simulink model "Demo_veDYNA_cs"  (Simulink 7.6)
settings: Solver=ode1  SolverMode=SingleTasking  StartTime=0  StopTime=15  FixedStep=1/500  RelTol=1e-3
PreLoadFcn:
  | PreScanveDYNAPreLoadFcn(bdroot);
  | check_NUTS_defined;
  | 
  | assignin('base',['model_closed_' bdroot],false);
PostLoadFcn:
  | PreScanveDYNAPostLoadFcn(bdroot);
  | 
InitFcn:
  | vdy_SetExternalInputSource('ManLongCtrl',1,'Brake','other');
  | vdy_SetExternalInputSource('ManLongCtrl',1,'EngineTorque','other');
  | vdy_SetExternalInputSource('ManLatCtrl',1,'Steering','other');
  | 
  | PreScanveDYNAInitFcn(bdroot);
  | PreScanExperimentInitFcn(bdroot)
StopFcn:
  | PreScanExperimentStopFcn(bdroot)
undefined symbols (not defined in the file): at_period, CPT, DiscIntNeverNeededParam, vm_at_pulsewidth, vm_driver_dflt_gain, x_ini_VRML, y_ini_VRML, z_ini_VRML
libraries: dyna_cpt_lib x93, PreScanSimulinkLibrary x10, PreScanUsefulBlocks x4, simulink x4, anilib x3, dyna_lib x3, simulink_extras x2, dyna_manctrl_lib x2, dyna_road_lib x2, dyna_io_lib x1, dyna_demo_lib x1, dyna_usr_maneuver_states_lib x1
(part 5 of 8)

== system Demo_veDYNA_cs/Mazda_RX8_1/Simple ACC/Engine Torque Control/Demux Vehicle Info/gear_ratio ==
  RStatF : Inport
  GearRatioF : Inport  Port=2
  RStatR : Inport  Port=3
  GearRatioR : Inport  Port=4
  Product1 : Product  Inputs=/*  SaturateOnIntegerOverflow=on  InputSameDT=on  OutDataTypeStr=Inherit: Same as first input
  Product2 : Product  Inputs=/*  SaturateOnIntegerOverflow=on  InputSameDT=on  OutDataTypeStr=Inherit: Same as first input
  Sum : Sum  Inputs=|++  SaturateOnIntegerOverflow=on  InputSameDT=on  OutDataTypeStr=Inherit: Same as first input
  GearRatio : Outport
  wires:
  Sum/1 -> GearRatio/1
  Product2/1 -> Sum/1
  Product1/1 -> Sum/2
  RStatF/1 -> Product2/1
  GearRatioF/1 -> Product2/2
  RStatR/1 -> Product1/1
  GearRatioR/1 -> Product1/2

== system Demo_veDYNA_cs/Mazda_RX8_1/Simple ACC/Engine Torque Control/Demux Vehicle Info/mmot diff ==
  vIst : Inport
  gear_ratio : Inport  Port=2
  Theta : Inport  Port=3
  Theta Mot : Inport  Port=4
  vSoll : Inport  Port=5
  Product : Product  Inputs=3  SaturateOnIntegerOverflow=on  InputSameDT=on  OutDataTypeStr=Inherit: Same as first input
  Sum : Sum  Inputs=|++  SaturateOnIntegerOverflow=on  InputSameDT=on  OutDataTypeStr=Inherit: Same as first input
  Sum1 : Sum  Inputs=+-  SaturateOnIntegerOverflow=on  InputSameDT=on  OutDataTypeStr=Inherit: Same as first input
  Out1 : Outport
  wires:
  Product/1 -> Out1/1
  Sum1/1 -> Product/1
  Sum/1 -> Product/3
  gear_ratio/1 -> Product/2
  vSoll/1 -> Sum1/1
  vIst/1 -> Sum1/2
  Theta/1 -> Sum/1
  Theta Mot/1 -> Sum/2

== system Demo_veDYNA_cs/Mazda_RX8_1/Simple ACC/Engine Torque Control/Demux Vehicle Info/theta_red ==
  gear ratio : Inport
  VehMass : Inport  Port=2
  Constant : Constant
  Math Function : Math  Operator=square  SaturateOnIntegerOverflow=on
  Product1 : Product  Inputs=/*  SaturateOnIntegerOverflow=on  InputSameDT=on  OutDataTypeStr=Inherit: Same as first input
  Sum : Sum  Inputs=++|  SaturateOnIntegerOverflow=on  InputSameDT=on  OutDataTypeStr=Inherit: Same as first input
  Theta : Outport
  wires:
  Constant/1 -> Sum/1
  Sum/1 -> Product1/1
  Math Function/1 -> Sum/2
  gear ratio/1 -> Math Function/1
  Product1/1 -> Theta/1
  VehMass/1 -> Product1/2

== system Demo_veDYNA_cs/Nissan_Cabstar_1/Trajectories/Traj2State1/Traj2State2/MuxState ==
  x [m] : Inport
  y [m] : Inport  Port=2
  z [m] : Inport  Port=3
  dx [m/s] : Inport  Port=4
  dy [m/s] : Inport  Port=5
  dz [m/s] : Inport  Port=6
  R [rad] : Inport  Port=7
  P [rad] : Inport  Port=8
  Y [rad] : Inport  Port=9
  Mux : Mux  Inputs=9
  state : Outport
  wires:
  z [m]/1 -> Mux/3
  y [m]/1 -> Mux/2
  x [m]/1 -> Mux/1
  Y [rad]/1 -> Mux/9
  P [rad]/1 -> Mux/8
  R [rad]/1 -> Mux/7
  dz [m/s]/1 -> Mux/6
  dy [m/s]/1 -> Mux/5
  dx [m/s]/1 -> Mux/4
  Mux/1 -> state/1

== system Demo_veDYNA_cs/Nissan_Cabstar_1/Trajectories/Traj2State1/Traj2State2/Traj2MuxState_Ext ==
  Traj : Inport
  Terminator{1..9} (9 alike) : Terminator
  demux : Subsystem
  x [m] : Outport
  y [m] : Outport  Port=2
  z [m] : Outport  Port=3
  dx [m/s] : Outport  Port=4
  dy [m/s] : Outport  Port=5
  dz [m/s] : Outport  Port=6
  R [rad] : Outport  Port=7
  P [rad] : Outport  Port=8
  Y [rad] : Outport  Port=9
  wires:
  demux/9(Y) -> Y [rad]/1
  demux/7(R) -> R [rad]/1
  demux/5(vely) -> dy [m/s]/1
  demux/4(velx) -> dx [m/s]/1
  demux/10(velR) -> Terminator4/1
  demux/11(velP) -> Terminator5/1
  demux/12(velY) -> Terminator1/1
  demux/13(accx) -> Terminator8/1
  demux/14(accy) -> Terminator9/1
  demux/15(accz) -> Terminator7/1
  demux/18(accY) -> Terminator2/1
  demux/16(accR) -> Terminator3/1
  demux/17(accP) -> Terminator6/1
  demux/3(z) -> z [m]/1
  Traj/1 -> demux/1(traj)
  demux/6(velz) -> dz [m/s]/1
  demux/1(x) -> x [m]/1
  demux/2(y) -> y [m]/1
  demux/8(P) -> P [rad]/1

== system Demo_veDYNA_cs/Vedyna_Vehicle/CPT_MDL/MDL_PAR/BrkHyd/System Instance 1 ==
  pbrmaster [N/m**2] : Subsystem
      mask Display: disp('Master brake cylinder pressure [N/m**2]')

== system Demo_veDYNA_cs/Vedyna_Vehicle/CPT_MDL/MDL_PAR/ClutchCtrl/System Instance 1 ==
  Clutch [%] : Subsystem
      mask Display: disp('Clutch ratio [%]')

== system Demo_veDYNA_cs/Vedyna_Vehicle/CPT_MDL/MDL_PAR/Contact/System Instance 1 ==
  RoadZ [m] : Subsystem
      mask Display: disp('Local road excitation [m]')

== system Demo_veDYNA_cs/Vedyna_Vehicle/CPT_MDL/MDL_PAR/Contact/System Instance 2 ==
  RoadZ [m] : Subsystem
      mask Display: disp('Local road excitation [m]')

== system Demo_veDYNA_cs/Vedyna_Vehicle/CPT_MDL/MDL_PAR/Contact/System Instance 3 ==
  RoadZ [m] : Subsystem
      mask Display: disp('Local road excitation [m]')

== system Demo_veDYNA_cs/Vedyna_Vehicle/CPT_MDL/MDL_PAR/Contact/System Instance 4 ==
  RoadZ [m] : Subsystem
      mask Display: disp('Local road excitation [m]')

== system Demo_veDYNA_cs/Vedyna_Vehicle/CPT_MDL/MDL_PAR/Contact/System Instance 5 ==
  RoadZ [m] : Subsystem
      mask Display: disp('Local road excitation [m]')

== system Demo_veDYNA_cs/Vedyna_Vehicle/CPT_MDL/MDL_PAR/Contact/System Instance 6 ==
  RoadZ [m] : Subsystem
      mask Display: disp('Local road excitation [m]')

== system Demo_veDYNA_cs/Vedyna_Vehicle/CPT_MDL/MDL_PAR/Contact/System Instance 7 ==
  RoadZ [m] : Subsystem
      mask Display: disp('Local road excitation [m]')

== system Demo_veDYNA_cs/Vedyna_Vehicle/CPT_MDL/MDL_PAR/Contact/System Instance 8 ==
  RoadZ [m] : Subsystem
      mask Display: disp('Local road excitation [m]')

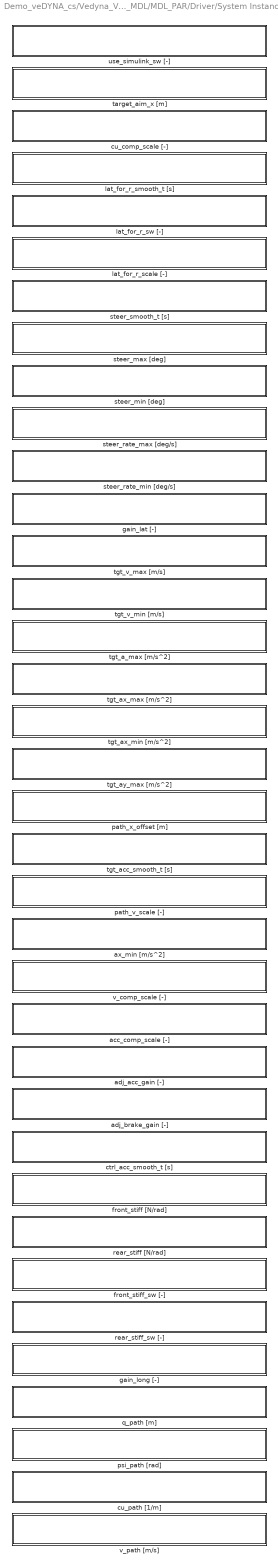
== system Demo_veDYNA_cs/Vedyna_Vehicle/CPT_MDL/MDL_PAR/Driver/System Instance 1 ==
  acc_comp_scale [-] : Subsystem
      mask Display: disp('v (acc_comp_scale) [-]')
  adj_acc_gain [-] : Subsystem
      mask Display: disp('v (adj_acc_gain) [-]')
  adj_brake_gain [-] : Subsystem
      mask Display: disp('v (adj_brake_gain) [-]')
  ax_min [m/s^2] : Subsystem
      mask Display: disp('v (ax_min) [m/s^2]')
  ctrl_acc_smooth_t [s] : Subsystem
      mask Display: disp('v (ctrl_acc_smooth_t) [s]')
  cu_comp_scale [-] : Subsystem
      mask Display: disp('v (cu_comp_scale) [-]')
  cu_path [1/m] : Subsystem
      mask Display: disp('path curvature [1/m]')
  front_stiff [N/rad] : Subsystem
      mask Display: disp('v (front_stiff) [N/rad]')
  front_stiff_sw [-] : Subsystem
      mask Display: disp('v (front_stiff_sw) [-]')
  gain_lat [-] : Subsystem
      mask Display: disp('v (gain_lat) [-]')
  gain_long [-] : Subsystem
      mask Display: disp('v (gain_long) [-]')
  lat_for_r_scale [-] : Subsystem
      mask Display: disp('v (lat_for_r_scale) [-]')
  lat_for_r_smooth_t [s] : Subsystem
      mask Display: disp('v (lat_for_r_smooth_t) [s]')
  lat_for_r_sw [-] : Subsystem
      mask Display: disp('v (lat_for_r_sw) [-]')
  path_v_scale [-] : Subsystem
      mask Display: disp('v (path_v_scale) [-]')
  path_x_offset [m] : Subsystem
      mask Display: disp('v (path_x_offset) [m]')
  psi_path [rad] : Subsystem
      mask Display: disp('path angle offset (relative to road''s center line) [rad]')
  q_path [m] : Subsystem
      mask Display: disp('lateral offset [m]')
  rear_stiff [N/rad] : Subsystem
      mask Display: disp('v (rear_stiff) [N/rad]')
  rear_stiff_sw [-] : Subsystem
      mask Display: disp('v (rear_stiff_sw) [-]')
  steer_max [deg] : Subsystem
      mask Display: disp('v (steer_max) [deg]')
  steer_min [deg] : Subsystem
      mask Display: disp('v (steer_min) [deg]')
  steer_rate_max [deg/s] : Subsystem
      mask Display: disp('v (steer_rate_max) [deg/s]')
  steer_rate_min [deg/s] : Subsystem
      mask Display: disp('v (steer_rate_min) [deg/s]')
  steer_smooth_t [s] : Subsystem
      mask Display: disp('v (steer_smooth_t) [s]')
  target_aim_x [m] : Subsystem
      mask Display: disp('v (target_aim_x) [m]')
  tgt_a_max [m/s^2] : Subsystem
      mask Display: disp('v (tgt_a_max) [m/s^2]')
  tgt_acc_smooth_t [s] : Subsystem
      mask Display: disp('v (tgt_acc_smooth_t) [s]')
  tgt_ax_max [m/s^2] : Subsystem
      mask Display: disp('v (tgt_ax_max) [m/s^2]')
  tgt_ax_min [m/s^2] : Subsystem
      mask Display: disp('v (tgt_ax_min) [m/s^2]')
  tgt_ay_max [m/s^2] : Subsystem
      mask Display: disp('v (tgt_ay_max) [m/s^2]')
  tgt_v_max [m/s] : Subsystem
      mask Display: disp('v (tgt_v_max) [m/s]')
  tgt_v_min [m/s] : Subsystem
      mask Display: disp('v (tgt_v_min) [m/s]')
  use_simulink_sw [-] : Subsystem
      mask Display: disp('v (use_simulink_sw) [-]')
  v_comp_scale [-] : Subsystem
      mask Display: disp('v (v_comp_scale) [-]')
  v_path [m/s] : Subsystem
      mask Display: disp('desired velocity [m/s]')

== system Demo_veDYNA_cs/Vedyna_Vehicle/CPT_MDL/MDL_PAR/Engine/System Instance 1 ==
  ASR_Flag [-] : Subsystem
      mask Display: disp('ASR Flag [-]')
  ASR_Torque [Nm] : Subsystem
      mask Display: disp('ASR Torque [Nm]')
  MSR_Flag [-] : Subsystem
      mask Display: disp('MSR Flag [-]')
  MSR_Torque [Nm] : Subsystem
      mask Display: disp('MSR Torque [Nm]')

== system Demo_veDYNA_cs/Vedyna_Vehicle/CPT_MDL/MDL_PAR/GearCtrl/System Instance 1 ==
  Gear [-] : Subsystem
      mask Display: disp('Gear position [-]')
  UpShiftRequest [-1,1] : Subsystem
      mask Display: disp('Up shift request [-1,1]')

== system Demo_veDYNA_cs/Vedyna_Vehicle/CPT_MDL/MDL_PAR/ManLatCtrl/System Instance 1 ==
  Curvature [1/m] : Subsystem
      mask Display: disp('Curvature [1/m]')
  Steering [deg] : Subsystem
      mask Display: disp('Steering wheel angle [deg]')

== system Demo_veDYNA_cs/Vedyna_Vehicle/CPT_MDL/MDL_PAR/ManLongCtrl/System Instance 1 ==
  AccelerationY [m/s**2] : Subsystem
      mask Display: disp('Lateral acceleration [m/s**2]')
  Brake [%] : Subsystem
      mask Display: disp('Brake position [%]')
  EngineTorque [Nm] : Subsystem
      mask Display: disp('Engine torque [Nm]')
  Speed [km/h] : Subsystem
      mask Display: disp('Speed [km/h]')
  Throttle [%] : Subsystem
      mask Display: disp('Throttle position [%]')

== system Demo_veDYNA_cs/Vedyna_Vehicle/CPT_MDL/MDL_PAR/Tmeasy/System Instance 1 ==
  RoadMueScale [0..1] : Subsystem
      mask Display: disp('Road mue scaling factor [0..1]')

== system Demo_veDYNA_cs/Vedyna_Vehicle/CPT_MDL/MDL_PAR/Tmeasy/System Instance 2 ==
  RoadMueScale [0..1] : Subsystem
      mask Display: disp('Road mue scaling factor [0..1]')

== system Demo_veDYNA_cs/Vedyna_Vehicle/CPT_MDL/MDL_PAR/Tmeasy/System Instance 3 ==
  RoadMueScale [0..1] : Subsystem
      mask Display: disp('Road mue scaling factor [0..1]')

== system Demo_veDYNA_cs/Vedyna_Vehicle/CPT_MDL/MDL_PAR/Tmeasy/System Instance 4 ==
  RoadMueScale [0..1] : Subsystem
      mask Display: disp('Road mue scaling factor [0..1]')

== system Demo_veDYNA_cs/Vedyna_Vehicle/CPT_MDL/MDL_PAR/Tmeasy/System Instance 5 ==
  RoadMueScale [0..1] : Subsystem
      mask Display: disp('Road mue scaling factor [0..1]')

== system Demo_veDYNA_cs/Vedyna_Vehicle/CPT_MDL/MDL_PAR/Tmeasy/System Instance 6 ==
  RoadMueScale [0..1] : Subsystem
      mask Display: disp('Road mue scaling factor [0..1]')

== system Demo_veDYNA_cs/Vedyna_Vehicle/CPT_MDL/MDL_PAR/Tmeasy/System Instance 7 ==
  RoadMueScale [0..1] : Subsystem
      mask Display: disp('Road mue scaling factor [0..1]')

== system Demo_veDYNA_cs/Vedyna_Vehicle/CPT_MDL/MDL_PAR/Tmeasy/System Instance 8 ==
  RoadMueScale [0..1] : Subsystem
      mask Display: disp('Road mue scaling factor [0..1]')

== system Demo_veDYNA_cs/Vedyna_Vehicle/CPT_MDL/MDL_PAR/Wheel/System Instance 1 ==
  pbrm [N/m**2] : Subsystem
      mask Display: disp('Wheel cylinder brake pressure [N/m**2]')

== system Demo_veDYNA_cs/Vedyna_Vehicle/CPT_MDL/MDL_PAR/Wheel/System Instance 2 ==
  pbrm [N/m**2] : Subsystem
      mask Display: disp('Wheel cylinder brake pressure [N/m**2]')

== system Demo_veDYNA_cs/Vedyna_Vehicle/CPT_MDL/MDL_PAR/Wheel/System Instance 3 ==
  pbrm [N/m**2] : Subsystem
      mask Display: disp('Wheel cylinder brake pressure [N/m**2]')

== system Demo_veDYNA_cs/Vedyna_Vehicle/CPT_MDL/MDL_PAR/Wheel/System Instance 4 ==
  pbrm [N/m**2] : Subsystem
      mask Display: disp('Wheel cylinder brake pressure [N/m**2]')

== system Demo_veDYNA_cs/Vedyna_Vehicle/CPT_MDL/MDL_PAR/Wheel/System Instance 5 ==
  pbrm [N/m**2] : Subsystem
      mask Display: disp('Wheel cylinder brake pressure [N/m**2]')

== system Demo_veDYNA_cs/Vedyna_Vehicle/CPT_MDL/MDL_PAR/Wheel/System Instance 6 ==
  pbrm [N/m**2] : Subsystem
      mask Display: disp('Wheel cylinder brake pressure [N/m**2]')

== system Demo_veDYNA_cs/Vedyna_Vehicle/CPT_MDL/MDL_PAR/Wheel/System Instance 7 ==
  pbrm [N/m**2] : Subsystem
      mask Display: disp('Wheel cylinder brake pressure [N/m**2]')

== system Demo_veDYNA_cs/Vedyna_Vehicle/CPT_MDL/MDL_PAR/Wheel/System Instance 8 ==
  pbrm [N/m**2] : Subsystem
      mask Display: disp('Wheel cylinder brake pressure [N/m**2]')

== system Demo_veDYNA_cs/Vedyna_Vehicle/CPT_MDL/MDL_SW/BrkHyd/System Instance 1 ==
  HCI [1,..,n] : Subsystem
      mask Display: disp('HCI switch [1,..,n]')
  pbrmaster [1,..,4] : Subsystem
      mask Display: disp('Input switch: value(1), table(2), io(3), other(4) [1,..,4]')

== system Demo_veDYNA_cs/Vedyna_Vehicle/CPT_MDL/MDL_SW/Chassis/System Instance 1 ==
  HCI [1,..,n] : Subsystem
      mask Display: disp('HCI switch [1,..,n]')

== system Demo_veDYNA_cs/Vedyna_Vehicle/CPT_MDL/MDL_SW/ClutchCtrl/System Instance 1 ==
  Clutch [1,..,4] : Subsystem
      mask Display: disp('Input switch: value(1), table(2), io(3), other(4) [1,..,4]')
  ClutchMode [0,1] : Subsystem
      mask Display: disp('Input switch: internal(0), external(1) [0,1]')
  HCI [1,..,n] : Subsystem
      mask Display: disp('HCI switch [1,..,n]')

== system Demo_veDYNA_cs/Vedyna_Vehicle/CPT_MDL/MDL_SW/Contact/System Instance 1 ==
  RoadZ [1,..,4] : Subsystem
      mask Display: disp('Input switch: value(1), table(2), io(3), other(4) [1,..,4]')

== system Demo_veDYNA_cs/Vedyna_Vehicle/CPT_MDL/MDL_SW/Contact/System Instance 2 ==
  RoadZ [1,..,4] : Subsystem
      mask Display: disp('Input switch: value(1), table(2), io(3), other(4) [1,..,4]')

== system Demo_veDYNA_cs/Vedyna_Vehicle/CPT_MDL/MDL_SW/Contact/System Instance 3 ==
  RoadZ [1,..,4] : Subsystem
      mask Display: disp('Input switch: value(1), table(2), io(3), other(4) [1,..,4]')

== system Demo_veDYNA_cs/Vedyna_Vehicle/CPT_MDL/MDL_SW/Contact/System Instance 4 ==
  RoadZ [1,..,4] : Subsystem
      mask Display: disp('Input switch: value(1), table(2), io(3), other(4) [1,..,4]')

== system Demo_veDYNA_cs/Vedyna_Vehicle/CPT_MDL/MDL_SW/Contact/System Instance 5 ==
  RoadZ [1,..,4] : Subsystem
      mask Display: disp('Input switch: value(1), table(2), io(3), other(4) [1,..,4]')

== system Demo_veDYNA_cs/Vedyna_Vehicle/CPT_MDL/MDL_SW/Contact/System Instance 6 ==
  RoadZ [1,..,4] : Subsystem
      mask Display: disp('Input switch: value(1), table(2), io(3), other(4) [1,..,4]')

== system Demo_veDYNA_cs/Vedyna_Vehicle/CPT_MDL/MDL_SW/Contact/System Instance 7 ==
  RoadZ [1,..,4] : Subsystem
      mask Display: disp('Input switch: value(1), table(2), io(3), other(4) [1,..,4]')

== system Demo_veDYNA_cs/Vedyna_Vehicle/CPT_MDL/MDL_SW/Contact/System Instance 8 ==
  RoadZ [1,..,4] : Subsystem
      mask Display: disp('Input switch: value(1), table(2), io(3), other(4) [1,..,4]')

== system Demo_veDYNA_cs/Vedyna_Vehicle/CPT_MDL/MDL_SW/Driveline/System Instance 1 ==
  HCI [1,..,n] : Subsystem
      mask Display: disp('HCI switch [1,..,n]')

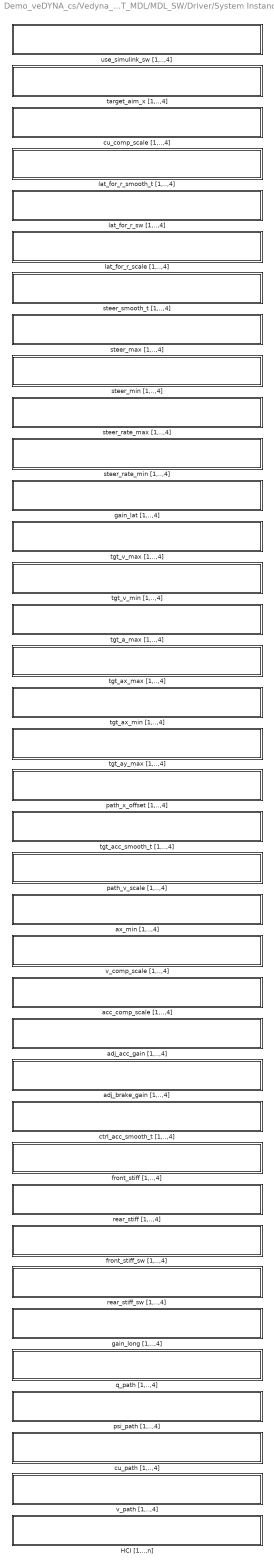
== system Demo_veDYNA_cs/Vedyna_Vehicle/CPT_MDL/MDL_SW/Driver/System Instance 1 ==
  HCI [1,..,n] : Subsystem
      mask Display: disp('HCI switch [1,..,n]')
  acc_comp_scale [1,..,4] : Subsystem
      mask Display: disp('Input switch: value(1), table(2), io(3), other(4) [1,..,4]')
  adj_acc_gain [1,..,4] : Subsystem
      mask Display: disp('Input switch: value(1), table(2), io(3), other(4) [1,..,4]')
  adj_brake_gain [1,..,4] : Subsystem
      mask Display: disp('Input switch: value(1), table(2), io(3), other(4) [1,..,4]')
  ax_min [1,..,4] : Subsystem
      mask Display: disp('Input switch: value(1), table(2), io(3), other(4) [1,..,4]')
  ctrl_acc_smooth_t [1,..,4] : Subsystem
      mask Display: disp('Input switch: value(1), table(2), io(3), other(4) [1,..,4]')
  cu_comp_scale [1,..,4] : Subsystem
      mask Display: disp('Input switch: value(1), table(2), io(3), other(4) [1,..,4]')
  cu_path [1,..,4] : Subsystem
      mask Display: disp('Input switch: value(1), table(2), io(3), other(4) [1,..,4]')
  front_stiff [1,..,4] : Subsystem
      mask Display: disp('Input switch: value(1), table(2), io(3), other(4) [1,..,4]')
  front_stiff_sw [1,..,4] : Subsystem
      mask Display: disp('Input switch: value(1), table(2), io(3), other(4) [1,..,4]')
  gain_lat [1,..,4] : Subsystem
      mask Display: disp('Input switch: value(1), table(2), io(3), other(4) [1,..,4]')
  gain_long [1,..,4] : Subsystem
      mask Display: disp('Input switch: value(1), table(2), io(3), other(4) [1,..,4]')
  lat_for_r_scale [1,..,4] : Subsystem
      mask Display: disp('Input switch: value(1), table(2), io(3), other(4) [1,..,4]')
  lat_for_r_smooth_t [1,..,4] : Subsystem
      mask Display: disp('Input switch: value(1), table(2), io(3), other(4) [1,..,4]')
  lat_for_r_sw [1,..,4] : Subsystem
      mask Display: disp('Input switch: value(1), table(2), io(3), other(4) [1,..,4]')
  path_v_scale [1,..,4] : Subsystem
      mask Display: disp('Input switch: value(1), table(2), io(3), other(4) [1,..,4]')
  path_x_offset [1,..,4] : Subsystem
      mask Display: disp('Input switch: value(1), table(2), io(3), other(4) [1,..,4]')
  psi_path [1,..,4] : Subsystem
      mask Display: disp('Input switch: value(1), table(2), io(3), other(4) [1,..,4]')
  q_path [1,..,4] : Subsystem
      mask Display: disp('Input switch: value(1), table(2), io(3), other(4) [1,..,4]')
  rear_stiff [1,..,4] : Subsystem
      mask Display: disp('Input switch: value(1), table(2), io(3), other(4) [1,..,4]')
  rear_stiff_sw [1,..,4] : Subsystem
      mask Display: disp('Input switch: value(1), table(2), io(3), other(4) [1,..,4]')
  steer_max [1,..,4] : Subsystem
      mask Display: disp('Input switch: value(1), table(2), io(3), other(4) [1,..,4]')
  steer_min [1,..,4] : Subsystem
      mask Display: disp('Input switch: value(1), table(2), io(3), other(4) [1,..,4]')
  steer_rate_max [1,..,4] : Subsystem
      mask Display: disp('Input switch: value(1), table(2), io(3), other(4) [1,..,4]')
  steer_rate_min [1,..,4] : Subsystem
      mask Display: disp('Input switch: value(1), table(2), io(3), other(4) [1,..,4]')
  steer_smooth_t [1,..,4] : Subsystem
      mask Display: disp('Input switch: value(1), table(2), io(3), other(4) [1,..,4]')
  target_aim_x [1,..,4] : Subsystem
      mask Display: disp('Input switch: value(1), table(2), io(3), other(4) [1,..,4]')
  tgt_a_max [1,..,4] : Subsystem
      mask Display: disp('Input switch: value(1), table(2), io(3), other(4) [1,..,4]')
  tgt_acc_smooth_t [1,..,4] : Subsystem
      mask Display: disp('Input switch: value(1), table(2), io(3), other(4) [1,..,4]')
  tgt_ax_max [1,..,4] : Subsystem
      mask Display: disp('Input switch: value(1), table(2), io(3), other(4) [1,..,4]')
  tgt_ax_min [1,..,4] : Subsystem
      mask Display: disp('Input switch: value(1), table(2), io(3), other(4) [1,..,4]')
  tgt_ay_max [1,..,4] : Subsystem
      mask Display: disp('Input switch: value(1), table(2), io(3), other(4) [1,..,4]')
  tgt_v_max [1,..,4] : Subsystem
      mask Display: disp('Input switch: value(1), table(2), io(3), other(4) [1,..,4]')
  tgt_v_min [1,..,4] : Subsystem
      mask Display: disp('Input switch: value(1), table(2), io(3), other(4) [1,..,4]')
  use_simulink_sw [1,..,4] : Subsystem
      mask Display: disp('Input switch: value(1), table(2), io(3), other(4) [1,..,4]')
  v_comp_scale [1,..,4] : Subsystem
      mask Display: disp('Input switch: value(1), table(2), io(3), other(4) [1,..,4]')
  v_path [1,..,4] : Subsystem
      mask Display: disp('Input switch: value(1), table(2), io(3), other(4) [1,..,4]')

== system Demo_veDYNA_cs/Vedyna_Vehicle/CPT_MDL/MDL_SW/Engine/System Instance 1 ==
  ASR_Flag [1,..,4] : Subsystem
      mask Display: disp('Input switch: value(1), table(2), io(3), other(4) [1,..,4]')
  ASR_Torque [1,..,4] : Subsystem
      mask Display: disp('Input switch: value(1), table(2), io(3), other(4) [1,..,4]')
  HCI [1,..,n] : Subsystem
      mask Display: disp('[Generated]')
  MSR_Flag [1,..,4] : Subsystem
      mask Display: disp('Input switch: value(1), table(2), io(3), other(4) [1,..,4]')
  MSR_Torque [1,..,4] : Subsystem
      mask Display: disp('Input switch: value(1), table(2), io(3), other(4) [1,..,4]')

== system Demo_veDYNA_cs/Vedyna_Vehicle/CPT_MDL/MDL_SW/GearCtrl/System Instance 1 ==
  Gear [1,..,4] : Subsystem
      mask Display: disp('Input switch: value(1), table(2), io(3), other(4) [1,..,4]')
  GearMode [0,1] : Subsystem
      mask Display: disp('Input switch: internal(0), external(1) [0,1]')
  HCI [1,..,n] : Subsystem
      mask Display: disp('HCI switch [1,..,n]')
  UpShiftRequest [1,..,4] : Subsystem
      mask Display: disp('Input switch: value(1), table(2), io(3), other(4) [1,..,4]')

== system Demo_veDYNA_cs/Vedyna_Vehicle/CPT_MDL/MDL_SW/ManLatCtrl/System Instance 1 ==
  Curvature [1,..,4] : Subsystem
      mask Display: disp('Input switch: value(1), table(2), io(3), other(4) [1,..,4]')
  LatManMode [0,1,2] : Subsystem
      mask Display: disp('Input switch: internal(0), ext. steering(1), ext. curvature(2) [0,1,2]')
  Steering [1,..,4] : Subsystem
      mask Display: disp('Input switch: value(1), table(2), io(3), other(4) [1,..,4]')

== system Demo_veDYNA_cs/Vedyna_Vehicle/CPT_MDL/MDL_SW/ManLongCtrl/System Instance 1 ==
  AccelerationY [1,..,4] : Subsystem
      mask Display: disp('Input switch: value(1), table(2), io(3), other(4) [1,..,4]')
  Brake [1,..,4] : Subsystem
      mask Display: disp('Input switch: value(1), table(2), io(3), other(4) [1,..,4]')
  EngineTorque [1,..,4] : Subsystem
      mask Display: disp('Input switch: value(1), table(2), io(3), other(4) [1,..,4]')
  LongManMode [0,1,2] : Subsystem
      mask Display: disp('Input switch: internal(0), ext. throttle/brake(1), ext. speed(2) [0,1,2]')
  Speed [1,..,4] : Subsystem
      mask Display: disp('Input switch: value(1), table(2), io(3), other(4) [1,..,4]')
  Throttle [1,..,4] : Subsystem
      mask Display: disp('Input switch: value(1), table(2), io(3), other(4) [1,..,4]')

== system Demo_veDYNA_cs/Vedyna_Vehicle/CPT_MDL/MDL_SW/ManSchedule/System Instance 1 ==
  HCI [1,..,n] : Subsystem
      mask Display: disp('HCI switch [1,..,n]')

== system Demo_veDYNA_cs/Vedyna_Vehicle/CPT_MDL/MDL_SW/ManSchedule/System Instance 2 ==
  HCI [1,..,n] : Subsystem
      mask Display: disp('HCI switch [1,..,n]')

== system Demo_veDYNA_cs/Vedyna_Vehicle/CPT_MDL/MDL_SW/ManSchedule/System Instance 3 ==
  HCI [1,..,n] : Subsystem
      mask Display: disp('HCI switch [1,..,n]')

== system Demo_veDYNA_cs/Vedyna_Vehicle/CPT_MDL/MDL_SW/Road/System Instance 1 ==
  HCI [1,..,n] : Subsystem
      mask Display: disp('HCI switch [1,..,n]')

== system Demo_veDYNA_cs/Vedyna_Vehicle/CPT_MDL/MDL_SW/Simctrl/System Instance 1 ==
  Reset [0,1] : Subsystem
      mask Display: disp('Reset switch: 0/1 [0,1]')
  Suspend [0,1] : Subsystem
      mask Display: disp('Suspend switch: 0/1 [0,1]')

== system Demo_veDYNA_cs/Vedyna_Vehicle/CPT_MDL/MDL_SW/Tmeasy/System Instance 1 ==
  HCI [1,..,n] : Subsystem
      mask Display: disp('HCI switch [1,..,n]')
  RoadMueScale [1,..,4] : Subsystem
      mask Display: disp('Input switch: value(1), table(2), io(3), other(4) [1,..,4]')

== system Demo_veDYNA_cs/Vedyna_Vehicle/CPT_MDL/MDL_SW/Tmeasy/System Instance 2 ==
  HCI [1,..,n] : Subsystem
      mask Display: disp('HCI switch [1,..,n]')
  RoadMueScale [1,..,4] : Subsystem
      mask Display: disp('Input switch: value(1), table(2), io(3), other(4) [1,..,4]')

== system Demo_veDYNA_cs/Vedyna_Vehicle/CPT_MDL/MDL_SW/Tmeasy/System Instance 3 ==
  HCI [1,..,n] : Subsystem
      mask Display: disp('HCI switch [1,..,n]')
  RoadMueScale [1,..,4] : Subsystem
      mask Display: disp('Input switch: value(1), table(2), io(3), other(4) [1,..,4]')

== system Demo_veDYNA_cs/Vedyna_Vehicle/CPT_MDL/MDL_SW/Tmeasy/System Instance 4 ==
  HCI [1,..,n] : Subsystem
      mask Display: disp('HCI switch [1,..,n]')
  RoadMueScale [1,..,4] : Subsystem
      mask Display: disp('Input switch: value(1), table(2), io(3), other(4) [1,..,4]')

== system Demo_veDYNA_cs/Vedyna_Vehicle/CPT_MDL/MDL_SW/Tmeasy/System Instance 5 ==
  HCI [1,..,n] : Subsystem
      mask Display: disp('HCI switch [1,..,n]')
  RoadMueScale [1,..,4] : Subsystem
      mask Display: disp('Input switch: value(1), table(2), io(3), other(4) [1,..,4]')

== system Demo_veDYNA_cs/Vedyna_Vehicle/CPT_MDL/MDL_SW/Tmeasy/System Instance 6 ==
  HCI [1,..,n] : Subsystem
      mask Display: disp('HCI switch [1,..,n]')
  RoadMueScale [1,..,4] : Subsystem
      mask Display: disp('Input switch: value(1), table(2), io(3), other(4) [1,..,4]')

== system Demo_veDYNA_cs/Vedyna_Vehicle/CPT_MDL/MDL_SW/Tmeasy/System Instance 7 ==
  HCI [1,..,n] : Subsystem
      mask Display: disp('HCI switch [1,..,n]')
  RoadMueScale [1,..,4] : Subsystem
      mask Display: disp('Input switch: value(1), table(2), io(3), other(4) [1,..,4]')

== system Demo_veDYNA_cs/Vedyna_Vehicle/CPT_MDL/MDL_SW/Tmeasy/System Instance 8 ==
  HCI [1,..,n] : Subsystem
      mask Display: disp('HCI switch [1,..,n]')
  RoadMueScale [1,..,4] : Subsystem
      mask Display: disp('Input switch: value(1), table(2), io(3), other(4) [1,..,4]')

== system Demo_veDYNA_cs/Vedyna_Vehicle/CPT_MDL/MDL_SW/Vehicle/System Instance 1 ==
  HCI [1,..,n] : Subsystem
      mask Display: disp('HCI switch [1,..,n]')

== system Demo_veDYNA_cs/Vedyna_Vehicle/CPT_MDL/MDL_SW/Wheel/System Instance 1 ==
  HCI [1,..,n] : Subsystem
      mask Display: disp('HCI switch [1,..,n]')
  pbrm [1,..,4] : Subsystem
      mask Display: disp('Input switch: value(1), table(2), io(3), other(4) [1,..,4]')

== system Demo_veDYNA_cs/Vedyna_Vehicle/CPT_MDL/MDL_SW/Wheel/System Instance 2 ==
  HCI [1,..,n] : Subsystem
      mask Display: disp('HCI switch [1,..,n]')
  pbrm [1,..,4] : Subsystem
      mask Display: disp('Input switch: value(1), table(2), io(3), other(4) [1,..,4]')

== system Demo_veDYNA_cs/Vedyna_Vehicle/CPT_MDL/MDL_SW/Wheel/System Instance 3 ==
  HCI [1,..,n] : Subsystem
      mask Display: disp('HCI switch [1,..,n]')
  pbrm [1,..,4] : Subsystem
      mask Display: disp('Input switch: value(1), table(2), io(3), other(4) [1,..,4]')

== system Demo_veDYNA_cs/Vedyna_Vehicle/CPT_MDL/MDL_SW/Wheel/System Instance 4 ==
  HCI [1,..,n] : Subsystem
      mask Display: disp('HCI switch [1,..,n]')
  pbrm [1,..,4] : Subsystem
      mask Display: disp('Input switch: value(1), table(2), io(3), other(4) [1,..,4]')

== system Demo_veDYNA_cs/Vedyna_Vehicle/CPT_MDL/MDL_SW/Wheel/System Instance 5 ==
  HCI [1,..,n] : Subsystem
      mask Display: disp('HCI switch [1,..,n]')
  pbrm [1,..,4] : Subsystem
      mask Display: disp('Input switch: value(1), table(2), io(3), other(4) [1,..,4]')

== system Demo_veDYNA_cs/Vedyna_Vehicle/CPT_MDL/MDL_SW/Wheel/System Instance 6 ==
  HCI [1,..,n] : Subsystem
      mask Display: disp('HCI switch [1,..,n]')
  pbrm [1,..,4] : Subsystem
      mask Display: disp('Input switch: value(1), table(2), io(3), other(4) [1,..,4]')

== system Demo_veDYNA_cs/Vedyna_Vehicle/CPT_MDL/MDL_SW/Wheel/System Instance 7 ==
  HCI [1,..,n] : Subsystem
      mask Display: disp('HCI switch [1,..,n]')
  pbrm [1,..,4] : Subsystem
      mask Display: disp('Input switch: value(1), table(2), io(3), other(4) [1,..,4]')

== system Demo_veDYNA_cs/Vedyna_Vehicle/CPT_MDL/MDL_SW/Wheel/System Instance 8 ==
  HCI [1,..,n] : Subsystem
      mask Display: disp('HCI switch [1,..,n]')
  pbrm [1,..,4] : Subsystem
      mask Display: disp('Input switch: value(1), table(2), io(3), other(4) [1,..,4]')

== system Demo_veDYNA_cs/Vedyna_Vehicle/vdy_mdl/Maneuver Control/Maneuver Controller Inputs/Clutch Control Inputs ==
  Ground : Ground
  Ground1 : Ground
  Mux : Mux  Inputs=2
  PAR_ClutchCtrl_1_Clutch : dyna_cpt_lib/CPT_MDL_PAR_ACCESS  Tag=vedynaCPT_MDL_PAR_ACCESS  component=ClutchCtrl  system_inst=1  parameter=Clutch
  SW_ClutchCtrl_1_ClutchMode : dyna_cpt_lib/CPT_MDL_SW_ACCESS  Tag=vedynaCPT_MDL_HCI_ACCESS  component=ClutchCtrl  system_inst=1  parameter=ClutchMode
  Scale to [0..1] : Gain  Gain=0.01  SaturateOnIntegerOverflow=on  OutDataTypeStr=Inherit: Same as input  ParamDataTypeStr=Inherit: Same as input
  Clutch Control Inputs : Outport
  wires:
  Scale to [0..1]/1 -> Mux/2
  PAR_ClutchCtrl_1_Clutch/1 -> Scale to [0..1]/1
  Ground1/1 -> PAR_ClutchCtrl_1_Clutch/1
  Ground/1 -> PAR_ClutchCtrl_1_Clutch/2
  SW_ClutchCtrl_1_ClutchMode/1 -> Mux/1
  Mux/1 -> Clutch Control Inputs/1

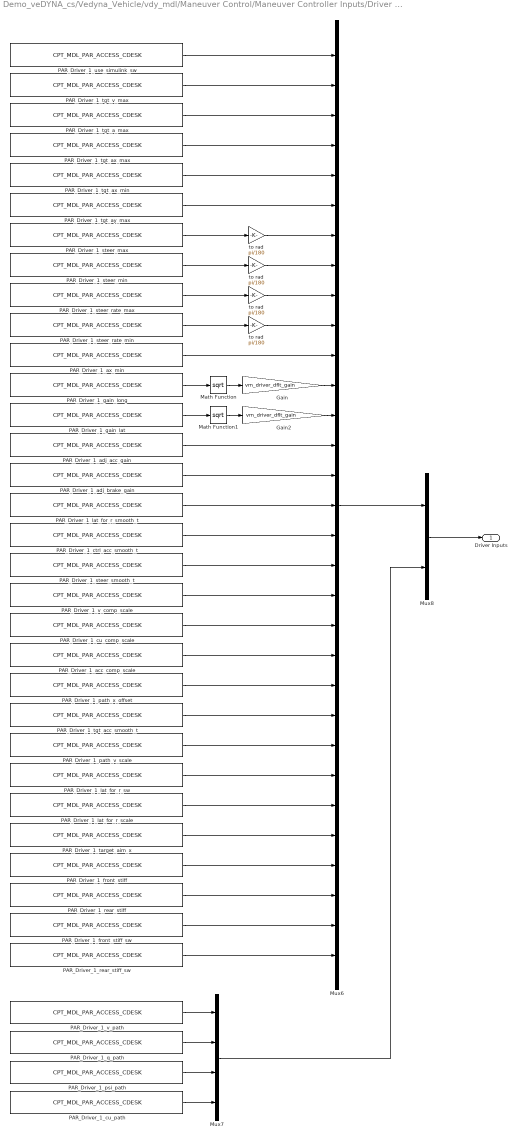
== system Demo_veDYNA_cs/Vedyna_Vehicle/vdy_mdl/Maneuver Control/Maneuver Controller Inputs/Driver Inputs ==
  Gain : Gain  Gain=vm_driver_dflt_gain  SaturateOnIntegerOverflow=on  OutDataTypeStr=Inherit: Same as input  ParamDataTypeStr=Inherit: Same as input
  Gain2 : Gain  Gain=vm_driver_dflt_gain  SaturateOnIntegerOverflow=on  OutDataTypeStr=Inherit: Same as input  ParamDataTypeStr=Inherit: Same as input
  Math Function : Math  Operator=sqrt  SaturateOnIntegerOverflow=on
  Math Function1 : Math  Operator=sqrt  SaturateOnIntegerOverflow=on
  Mux6 : Mux  Inputs=31
  Mux7 : Mux
  Mux8 : Mux  Inputs=2
  PAR_Driver_1_acc_comp_scale : dyna_cpt_lib/CPT_MDL_PAR_ACCESS_CDESK  Tag=vedynaCPT_MDL_PAR_ACCESS  component=Driver  system_inst=1  parameter=acc_comp_scale
  PAR_Driver_1_adj_acc_gain : dyna_cpt_lib/CPT_MDL_PAR_ACCESS_CDESK  Tag=vedynaCPT_MDL_PAR_ACCESS  component=Driver  system_inst=1  parameter=adj_acc_gain
  PAR_Driver_1_adj_brake_gain : dyna_cpt_lib/CPT_MDL_PAR_ACCESS_CDESK  Tag=vedynaCPT_MDL_PAR_ACCESS  component=Driver  system_inst=1  parameter=adj_brake_gain
  PAR_Driver_1_ax_min : dyna_cpt_lib/CPT_MDL_PAR_ACCESS_CDESK  Tag=vedynaCPT_MDL_PAR_ACCESS  component=Driver  system_inst=1  parameter=ax_min
  PAR_Driver_1_ctrl_acc_smooth_t : dyna_cpt_lib/CPT_MDL_PAR_ACCESS_CDESK  Tag=vedynaCPT_MDL_PAR_ACCESS  component=Driver  system_inst=1  parameter=ctrl_acc_smooth_t
  PAR_Driver_1_cu_comp_scale : dyna_cpt_lib/CPT_MDL_PAR_ACCESS_CDESK  Tag=vedynaCPT_MDL_PAR_ACCESS  component=Driver  system_inst=1  parameter=cu_comp_scale
  PAR_Driver_1_cu_path : dyna_cpt_lib/CPT_MDL_PAR_ACCESS_CDESK  Tag=vedynaCPT_MDL_PAR_ACCESS  component=Driver  system_inst=1  parameter=cu_path
  PAR_Driver_1_front_stiff : dyna_cpt_lib/CPT_MDL_PAR_ACCESS_CDESK  Tag=vedynaCPT_MDL_PAR_ACCESS  component=Driver  system_inst=1  parameter=front_stiff
  PAR_Driver_1_front_stiff_sw : dyna_cpt_lib/CPT_MDL_PAR_ACCESS_CDESK  Tag=vedynaCPT_MDL_PAR_ACCESS  component=Driver  system_inst=1  parameter=front_stiff_sw
  PAR_Driver_1_gain_lat : dyna_cpt_lib/CPT_MDL_PAR_ACCESS_CDESK  Tag=vedynaCPT_MDL_PAR_ACCESS  component=Driver  system_inst=1  parameter=gain_lat
  PAR_Driver_1_gain_long : dyna_cpt_lib/CPT_MDL_PAR_ACCESS_CDESK  Tag=vedynaCPT_MDL_PAR_ACCESS  component=Driver  system_inst=1  parameter=gain_long
  PAR_Driver_1_lat_for_r_scale : dyna_cpt_lib/CPT_MDL_PAR_ACCESS_CDESK  Tag=vedynaCPT_MDL_PAR_ACCESS  component=Driver  system_inst=1  parameter=lat_for_r_scale
  PAR_Driver_1_lat_for_r_smooth_t : dyna_cpt_lib/CPT_MDL_PAR_ACCESS_CDESK  Tag=vedynaCPT_MDL_PAR_ACCESS  component=Driver  system_inst=1  parameter=lat_for_r_smooth_t
  PAR_Driver_1_lat_for_r_sw : dyna_cpt_lib/CPT_MDL_PAR_ACCESS_CDESK  Tag=vedynaCPT_MDL_PAR_ACCESS  component=Driver  system_inst=1  parameter=lat_for_r_sw
  PAR_Driver_1_path_v_scale : dyna_cpt_lib/CPT_MDL_PAR_ACCESS_CDESK  Tag=vedynaCPT_MDL_PAR_ACCESS  component=Driver  system_inst=1  parameter=path_v_scale
  PAR_Driver_1_path_x_offset : dyna_cpt_lib/CPT_MDL_PAR_ACCESS_CDESK  Tag=vedynaCPT_MDL_PAR_ACCESS  component=Driver  system_inst=1  parameter=path_x_offset
  PAR_Driver_1_psi_path : dyna_cpt_lib/CPT_MDL_PAR_ACCESS_CDESK  Tag=vedynaCPT_MDL_PAR_ACCESS  component=Driver  system_inst=1  parameter=psi_path
  PAR_Driver_1_q_path : dyna_cpt_lib/CPT_MDL_PAR_ACCESS_CDESK  Tag=vedynaCPT_MDL_PAR_ACCESS  component=Driver  system_inst=1  parameter=q_path
  PAR_Driver_1_rear_stiff : dyna_cpt_lib/CPT_MDL_PAR_ACCESS_CDESK  Tag=vedynaCPT_MDL_PAR_ACCESS  component=Driver  system_inst=1  parameter=rear_stiff
  PAR_Driver_1_rear_stiff_sw : dyna_cpt_lib/CPT_MDL_PAR_ACCESS_CDESK  Tag=vedynaCPT_MDL_PAR_ACCESS  component=Driver  system_inst=1  parameter=rear_stiff_sw
  PAR_Driver_1_steer_max : dyna_cpt_lib/CPT_MDL_PAR_ACCESS_CDESK  Tag=vedynaCPT_MDL_PAR_ACCESS  component=Driver  system_inst=1  parameter=steer_max
  PAR_Driver_1_steer_min : dyna_cpt_lib/CPT_MDL_PAR_ACCESS_CDESK  Tag=vedynaCPT_MDL_PAR_ACCESS  component=Driver  system_inst=1  parameter=steer_min
  PAR_Driver_1_steer_rate_max : dyna_cpt_lib/CPT_MDL_PAR_ACCESS_CDESK  Tag=vedynaCPT_MDL_PAR_ACCESS  component=Driver  system_inst=1  parameter=steer_rate_max
  PAR_Driver_1_steer_rate_min : dyna_cpt_lib/CPT_MDL_PAR_ACCESS_CDESK  Tag=vedynaCPT_MDL_PAR_ACCESS  component=Driver  system_inst=1  parameter=steer_rate_min
  PAR_Driver_1_steer_smooth_t : dyna_cpt_lib/CPT_MDL_PAR_ACCESS_CDESK  Tag=vedynaCPT_MDL_PAR_ACCESS  component=Driver  system_inst=1  parameter=steer_smooth_t
  PAR_Driver_1_target_aim_x : dyna_cpt_lib/CPT_MDL_PAR_ACCESS_CDESK  Tag=vedynaCPT_MDL_PAR_ACCESS  component=Driver  system_inst=1  parameter=target_aim_x
  PAR_Driver_1_tgt_a_max : dyna_cpt_lib/CPT_MDL_PAR_ACCESS_CDESK  Tag=vedynaCPT_MDL_PAR_ACCESS  component=Driver  system_inst=1  parameter=tgt_a_max
  PAR_Driver_1_tgt_acc_smooth_t : dyna_cpt_lib/CPT_MDL_PAR_ACCESS_CDESK  Tag=vedynaCPT_MDL_PAR_ACCESS  component=Driver  system_inst=1  parameter=tgt_acc_smooth_t
  PAR_Driver_1_tgt_ax_max : dyna_cpt_lib/CPT_MDL_PAR_ACCESS_CDESK  Tag=vedynaCPT_MDL_PAR_ACCESS  component=Driver  system_inst=1  parameter=tgt_ax_max
  PAR_Driver_1_tgt_ax_min : dyna_cpt_lib/CPT_MDL_PAR_ACCESS_CDESK  Tag=vedynaCPT_MDL_PAR_ACCESS  component=Driver  system_inst=1  parameter=tgt_ax_min
  PAR_Driver_1_tgt_ay_max : dyna_cpt_lib/CPT_MDL_PAR_ACCESS_CDESK  Tag=vedynaCPT_MDL_PAR_ACCESS  component=Driver  system_inst=1  parameter=tgt_ay_max
  PAR_Driver_1_tgt_v_max : dyna_cpt_lib/CPT_MDL_PAR_ACCESS_CDESK  Tag=vedynaCPT_MDL_PAR_ACCESS  component=Driver  system_inst=1  parameter=tgt_v_max
  PAR_Driver_1_use_simulink_sw : dyna_cpt_lib/CPT_MDL_PAR_ACCESS_CDESK  Tag=vedynaCPT_MDL_PAR_ACCESS  component=Driver  system_inst=1  parameter=use_simulink_sw
  PAR_Driver_1_v_comp_scale : dyna_cpt_lib/CPT_MDL_PAR_ACCESS_CDESK  Tag=vedynaCPT_MDL_PAR_ACCESS  component=Driver  system_inst=1  parameter=v_comp_scale
  PAR_Driver_1_v_path : dyna_cpt_lib/CPT_MDL_PAR_ACCESS_CDESK  Tag=vedynaCPT_MDL_PAR_ACCESS  component=Driver  system_inst=1  parameter=v_path
  to rad : Gain  Gain=pi/180  SaturateOnIntegerOverflow=on  OutDataTypeStr=Inherit: Same as input  ParamDataTypeStr=Inherit: Same as input
  "to rad " : Gain  Gain=pi/180  SaturateOnIntegerOverflow=on  OutDataTypeStr=Inherit: Same as input  ParamDataTypeStr=Inherit: Same as input
  "to rad  " : Gain  Gain=pi/180  SaturateOnIntegerOverflow=on  OutDataTypeStr=Inherit: Same as input  ParamDataTypeStr=Inherit: Same as input
  "to rad   " : Gain  Gain=pi/180  SaturateOnIntegerOverflow=on  OutDataTypeStr=Inherit: Same as input  ParamDataTypeStr=Inherit: Same as input
  Driver Inputs : Outport
  wires:
  to rad/1 -> Mux6/7
  PAR_Driver_1_steer_max/1 -> to rad/1
  "to rad "/1 -> Mux6/8
  PAR_Driver_1_steer_min/1 -> "to rad "/1
  "to rad  "/1 -> Mux6/9
  PAR_Driver_1_steer_rate_max/1 -> "to rad  "/1
  "to rad   "/1 -> Mux6/10
  PAR_Driver_1_steer_rate_min/1 -> "to rad   "/1
  Math Function1/1 -> Gain2/1
  PAR_Driver_1_gain_lat/1 -> Math Function1/1
  Math Function/1 -> Gain/1
  PAR_Driver_1_gain_long/1 -> Math Function/1
  Gain2/1 -> Mux6/13
  Gain/1 -> Mux6/12
  Mux7/1 -> Mux8/2
  Mux8/1 -> Driver Inputs/1
  Mux6/1 -> Mux8/1
  PAR_Driver_1_cu_path/1 -> Mux7/4
  PAR_Driver_1_psi_path/1 -> Mux7/3
  PAR_Driver_1_q_path/1 -> Mux7/2
  PAR_Driver_1_v_path/1 -> Mux7/1
  PAR_Driver_1_rear_stiff_sw/1 -> Mux6/31
  PAR_Driver_1_front_stiff_sw/1 -> Mux6/30
  PAR_Driver_1_rear_stiff/1 -> Mux6/29
  PAR_Driver_1_front_stiff/1 -> Mux6/28
  PAR_Driver_1_target_aim_x/1 -> Mux6/27
  PAR_Driver_1_lat_for_r_scale/1 -> Mux6/26
  PAR_Driver_1_lat_for_r_sw/1 -> Mux6/25
  PAR_Driver_1_path_v_scale/1 -> Mux6/24
  PAR_Driver_1_tgt_acc_smooth_t/1 -> Mux6/23
  PAR_Driver_1_path_x_offset/1 -> Mux6/22
  PAR_Driver_1_acc_comp_scale/1 -> Mux6/21
  PAR_Driver_1_cu_comp_scale/1 -> Mux6/20
  PAR_Driver_1_v_comp_scale/1 -> Mux6/19
  PAR_Driver_1_steer_smooth_t/1 -> Mux6/18
  PAR_Driver_1_ctrl_acc_smooth_t/1 -> Mux6/17
  PAR_Driver_1_lat_for_r_smooth_t/1 -> Mux6/16
  PAR_Driver_1_adj_brake_gain/1 -> Mux6/15
  PAR_Driver_1_adj_acc_gain/1 -> Mux6/14
  PAR_Driver_1_ax_min/1 -> Mux6/11
  PAR_Driver_1_tgt_ay_max/1 -> Mux6/6
  PAR_Driver_1_tgt_ax_min/1 -> Mux6/5
  PAR_Driver_1_tgt_ax_max/1 -> Mux6/4
  PAR_Driver_1_tgt_a_max/1 -> Mux6/3
  PAR_Driver_1_tgt_v_max/1 -> Mux6/2
  PAR_Driver_1_use_simulink_sw/1 -> Mux6/1

== system Demo_veDYNA_cs/Vedyna_Vehicle/vdy_mdl/Maneuver Control/Maneuver Controller Inputs/Gear Control Inputs ==
  Ground{,1..3} (4 alike) : Ground
  Mux : Mux  Inputs=3
  PAR_GearCtrl_1_Gear : dyna_cpt_lib/CPT_MDL_PAR_ACCESS  Tag=vedynaCPT_MDL_PAR_ACCESS  component=GearCtrl  system_inst=1  parameter=Gear
  PAR_GearCtrl_1_UpShiftRequest : dyna_cpt_lib/CPT_MDL_PAR_ACCESS  Tag=vedynaCPT_MDL_PAR_ACCESS  component=GearCtrl  system_inst=1  parameter=UpShiftRequest
  SW_GearCtrl_1_GearMode : dyna_cpt_lib/CPT_MDL_SW_ACCESS  Tag=vedynaCPT_MDL_HCI_ACCESS  component=GearCtrl  system_inst=1  parameter=GearMode
  Gear Control Inputs : Outport
  wires:
  Ground1/1 -> PAR_GearCtrl_1_Gear/1
  Ground/1 -> PAR_GearCtrl_1_Gear/2
  SW_GearCtrl_1_GearMode/1 -> Mux/1
  PAR_GearCtrl_1_Gear/1 -> Mux/2
  PAR_GearCtrl_1_UpShiftRequest/1 -> Mux/3
  Ground3/1 -> PAR_GearCtrl_1_UpShiftRequest/1
  Ground2/1 -> PAR_GearCtrl_1_UpShiftRequest/2
  Mux/1 -> Gear Control Inputs/1

== system Demo_veDYNA_cs/Vedyna_Vehicle/vdy_mdl/Maneuver Control/Maneuver Controller Inputs/Lateral Control Inputs ==
  Ground{,1..3} (4 alike) : Ground
  Mux : Mux  Inputs=3
  PAR_ManLatCtrl_1_Curvature : dyna_cpt_lib/CPT_MDL_PAR_ACCESS  Tag=vedynaCPT_MDL_PAR_ACCESS  component=ManLatCtrl  system_inst=1  parameter=Curvature
  PAR_ManLatCtrl_1_Steering : dyna_cpt_lib/CPT_MDL_PAR_ACCESS  Tag=vedynaCPT_MDL_PAR_ACCESS  component=ManLatCtrl  system_inst=1  parameter=Steering
  SW_ManLatCtrl_1_LatManMode : dyna_cpt_lib/CPT_MDL_SW_ACCESS  Tag=vedynaCPT_MDL_HCI_ACCESS  component=ManLatCtrl  system_inst=1  parameter=LatManMode
  Scale to [rad] : Gain  Gain=pi/180  SaturateOnIntegerOverflow=on  OutDataTypeStr=Inherit: Same as input  ParamDataTypeStr=Inherit: Same as input
  Lateral Control Inputs : Outport
  wires:
  Scale to [rad]/1 -> Mux/2
  PAR_ManLatCtrl_1_Steering/1 -> Scale to [rad]/1
  SW_ManLatCtrl_1_LatManMode/1 -> Mux/1
  PAR_ManLatCtrl_1_Curvature/1 -> Mux/3
  Ground1/1 -> PAR_ManLatCtrl_1_Steering/1
  Ground/1 -> PAR_ManLatCtrl_1_Steering/2
  Ground3/1 -> PAR_ManLatCtrl_1_Curvature/1
  Ground2/1 -> PAR_ManLatCtrl_1_Curvature/2
  Mux/1 -> Lateral Control Inputs/1

== system Demo_veDYNA_cs/Vedyna_Vehicle/vdy_mdl/Maneuver Control/Maneuver Controller Inputs/Longitudinal Control Inputs ==
  Ground{,1..9} (10 alike) : Ground
  Mux : Mux  Inputs=6
  PAR_ManLongCtrl_1_AccelerationY : dyna_cpt_lib/CPT_MDL_PAR_ACCESS  Tag=vedynaCPT_MDL_PAR_ACCESS  component=ManLongCtrl  system_inst=1  parameter=AccelerationY
  PAR_ManLongCtrl_1_Brake : dyna_cpt_lib/CPT_MDL_PAR_ACCESS  Tag=vedynaCPT_MDL_PAR_ACCESS  component=ManLongCtrl  system_inst=1  parameter=Brake
  PAR_ManLongCtrl_1_EngineTorque : dyna_cpt_lib/CPT_MDL_PAR_ACCESS  Tag=vedynaCPT_MDL_PAR_ACCESS  component=ManLongCtrl  system_inst=1  parameter=EngineTorque
  PAR_ManLongCtrl_1_Speed : dyna_cpt_lib/CPT_MDL_PAR_ACCESS  Tag=vedynaCPT_MDL_PAR_ACCESS  component=ManLongCtrl  system_inst=1  parameter=Speed
  PAR_ManLongCtrl_1_Throttle : dyna_cpt_lib/CPT_MDL_PAR_ACCESS  Tag=vedynaCPT_MDL_PAR_ACCESS  component=ManLongCtrl  system_inst=1  parameter=Throttle
  SW_ManLongCtrl_1_LongManMode : dyna_cpt_lib/CPT_MDL_SW_ACCESS  Tag=vedynaCPT_MDL_HCI_ACCESS  component=ManLongCtrl  system_inst=1  parameter=LongManMode
  Scale to [0..1] : Gain  Gain=0.01  SaturateOnIntegerOverflow=on  OutDataTypeStr=Inherit: Same as input  ParamDataTypeStr=Inherit: Same as input
  Scale to [0..1]1 : Gain  Gain=0.01  SaturateOnIntegerOverflow=on  OutDataTypeStr=Inherit: Same as input  ParamDataTypeStr=Inherit: Same as input
  Scale to [m/s] : Gain  Gain=1/3.6  SaturateOnIntegerOverflow=on  OutDataTypeStr=Inherit: Same as input  ParamDataTypeStr=Inherit: Same as input
  Longitudinal Control Inputs : Outport
  wires:
  Scale to [m/s]/1 -> Mux/5
  PAR_ManLongCtrl_1_Speed/1 -> Scale to [m/s]/1
  Scale to [0..1]1/1 -> Mux/3
  PAR_ManLongCtrl_1_Brake/1 -> Scale to [0..1]1/1
  Scale to [0..1]/1 -> Mux/2
  PAR_ManLongCtrl_1_Throttle/1 -> Scale to [0..1]/1
  Ground1/1 -> PAR_ManLongCtrl_1_Throttle/1
  Ground/1 -> PAR_ManLongCtrl_1_Throttle/2
  SW_ManLongCtrl_1_LongManMode/1 -> Mux/1
  PAR_ManLongCtrl_1_AccelerationY/1 -> Mux/4
  PAR_ManLongCtrl_1_EngineTorque/1 -> Mux/6
  Ground9/1 -> PAR_ManLongCtrl_1_EngineTorque/1
  Ground8/1 -> PAR_ManLongCtrl_1_EngineTorque/2
  Ground7/1 -> PAR_ManLongCtrl_1_Speed/1
  Ground6/1 -> PAR_ManLongCtrl_1_Speed/2
  Ground5/1 -> PAR_ManLongCtrl_1_AccelerationY/1
  Ground4/1 -> PAR_ManLongCtrl_1_AccelerationY/2
  Ground3/1 -> PAR_ManLongCtrl_1_Brake/1
  Ground2/1 -> PAR_ManLongCtrl_1_Brake/2
  Mux/1 -> Longitudinal Control Inputs/1

== system Demo_veDYNA_cs/Vedyna_Vehicle/vdy_mdl/Road/veDYNA Road Subsystem/HCI Switch ==
  SW_Road_1_HCI : dyna_cpt_lib/CPT_MDL_HCI_SW_ACCESS  Tag=vedynaCPT_MDL_HCI_SW_ACCESS  component=Road  system_inst=1  parameter=HCI
  HCI Switch : Outport
  wires:
  SW_Road_1_HCI/1 -> HCI Switch/1

== system Demo_veDYNA_cs/Vedyna_Vehicle/vdy_mdl/Vehicle System/veDYNA Vehicle Subsystem/Brake System ==
  note: COPYRIGHT 2004 by TESIS DYNAware GmbH
  note: veDYNA Vehicle Brake System
  SyncIn : Inport
  I/O Vector : Inport  Port=2
  Brake Pedal Position : Inport  Port=3
  Configurable Subsystem : Subsystem  BlockChoice=veDYNA Brake Hydraulics
      settings: AttributesFormatString=%<BlockChoice>  MemberBlocks=User Defined Brake Hydraulics,veDYNA Brake Hydraulics,veDYNA Brake Hydraulics Trailer
      settings: TemplateBlock=|
      | dyna_brakehydraulics_lib/Configurable
      | Subsystem
  Constant{,1..5} (6 alike) : Constant  Value=0
  HCI Switch : Subsystem
  Mux1 : Mux  Inputs=6
  PAR_Wheel_1_pbrm : dyna_cpt_lib/CPT_MDL_PAR_ACCESS  Tag=vedynaCPT_MDL_PAR_ACCESS  component=Wheel  system_inst=1  parameter=pbrm
  PAR_Wheel_2_pbrm : dyna_cpt_lib/CPT_MDL_PAR_ACCESS  Tag=vedynaCPT_MDL_PAR_ACCESS  component=Wheel  system_inst=2  parameter=pbrm
  PAR_Wheel_3_pbrm : dyna_cpt_lib/CPT_MDL_PAR_ACCESS  Tag=vedynaCPT_MDL_PAR_ACCESS  component=Wheel  system_inst=3  parameter=pbrm
  PAR_Wheel_4_pbrm : dyna_cpt_lib/CPT_MDL_PAR_ACCESS  Tag=vedynaCPT_MDL_PAR_ACCESS  component=Wheel  system_inst=4  parameter=pbrm
  PAR_Wheel_5_pbrm : dyna_cpt_lib/CPT_MDL_PAR_ACCESS  Tag=vedynaCPT_MDL_PAR_ACCESS  component=Wheel  system_inst=5  parameter=pbrm
  PAR_Wheel_6_pbrm : dyna_cpt_lib/CPT_MDL_PAR_ACCESS  Tag=vedynaCPT_MDL_PAR_ACCESS  component=Wheel  system_inst=6  parameter=pbrm
  Terminator10 : Terminator
  Terminator4 : Terminator
  Brake Hydraulics Info : Outport
  SyncOut : Outport  Port=2
  Master Cylinder Pressure : Outport  Port=3
  Wheel Cylinder Pressures : Outport  Port=4
  tag scope: pb=global, pbmax=global
  wires:
  Configurable Subsystem/11(Wheel 8 Cylinder Pressure) -> Terminator10/1
  Configurable Subsystem/10(Wheel 7 Cylinder Pressure) -> Terminator4/1
  I/O Vector/1 -> Configurable Subsystem/2(I/O Vector)
  PAR_Wheel_2_pbrm/1 -> Mux1/2
  PAR_Wheel_3_pbrm/1 -> Mux1/3
  PAR_Wheel_4_pbrm/1 -> Mux1/4
  Mux1/1 -> Wheel Cylinder Pressures/1
  SyncIn/1 -> Configurable Subsystem/3(SyncIn)
  Brake Pedal Position/1 -> Configurable Subsystem/1(Brake Pedal Position)
  PAR_Wheel_1_pbrm/1 -> Mux1/1
  Configurable Subsystem/1(SyncOut) -> SyncOut/1
  Configurable Subsystem/2(BrkHyd Info) -> Brake Hydraulics Info/1, [pbmax]
  Configurable Subsystem/3(Master Cylinder Pressure) -> Master Cylinder Pressure/1, [pb]
  PAR_Wheel_5_pbrm/1 -> Mux1/5
  PAR_Wheel_6_pbrm/1 -> Mux1/6
  HCI Switch/1(HCI Switch) -> Configurable Subsystem/4(HCI Switch)
  Constant/1 -> PAR_Wheel_1_pbrm/1
  Configurable Subsystem/4(Wheel 1 Cylinder Pressure) -> PAR_Wheel_1_pbrm/2
  Configurable Subsystem/5(Wheel 2 Cylinder Pressure) -> PAR_Wheel_2_pbrm/2
  Configurable Subsystem/6(Wheel 3 Cylinder Pressure) -> PAR_Wheel_3_pbrm/2
  Configurable Subsystem/7(Wheel 4 Cylinder Pressure) -> PAR_Wheel_4_pbrm/2
  Configurable Subsystem/8(Wheel 5 Cylinder Pressure) -> PAR_Wheel_5_pbrm/2
  Configurable Subsystem/9(Wheel 6 Cylinder Pressure) -> PAR_Wheel_6_pbrm/2
  Constant1/1 -> PAR_Wheel_2_pbrm/1
  Constant2/1 -> PAR_Wheel_3_pbrm/1
  Constant3/1 -> PAR_Wheel_4_pbrm/1
  Constant4/1 -> PAR_Wheel_5_pbrm/1
  Constant5/1 -> PAR_Wheel_6_pbrm/1
